simulink model "sampleModel1927"  (R2023a)
settings: Solver=VariableStepAuto  StartTime=0.0  StopTime=10.0  RelTol=1e-3
libraries: hdlsllib x7, simulink x2
settings Model: Creator=user1  LastModifiedBy=user1

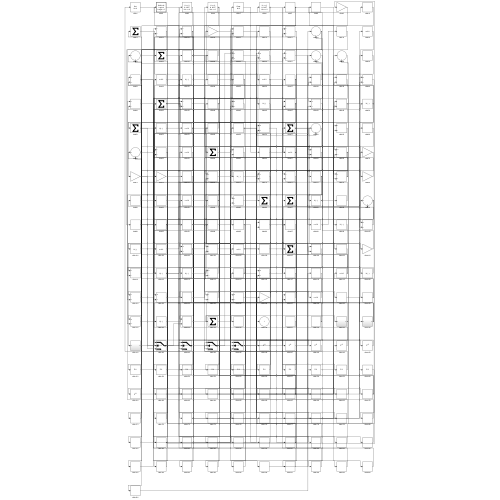
[thumbnail: Simulink's stored preview of the top-level diagram]
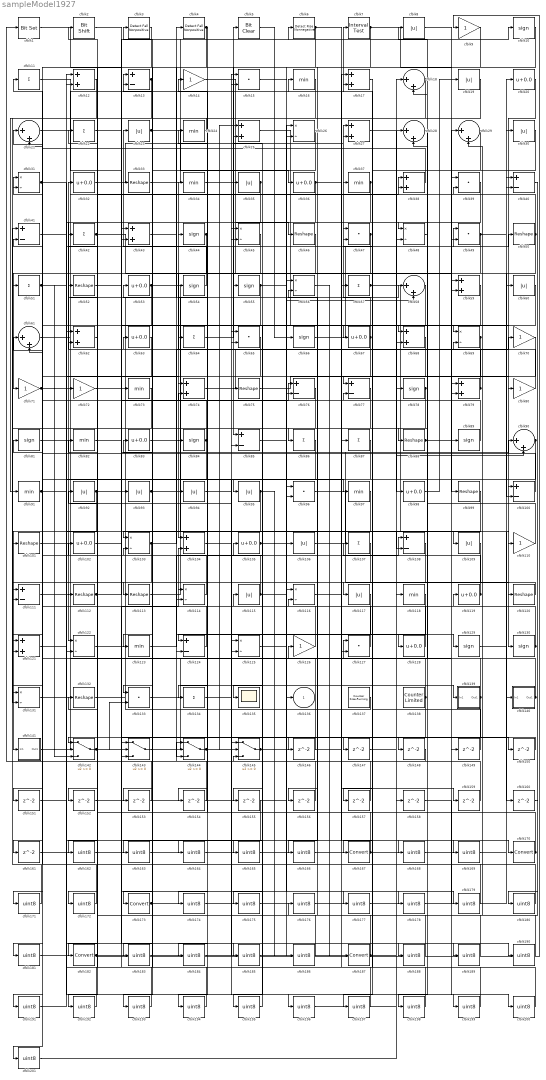
== system sampleModel1927 ==
  cfblk1 : simulink/Logic and Bit Operations/Bit Set  iBit=0
      settings: LibrarySourceBlock=|
      | hdlsllib/Logic and Bit
      | Operations/Bit Set
  cfblk{10,44,54..55,66,78,81,84,89,129..130} (11 alike) : Signum
  cfblk{13,40..41,76..77,85,100,108,111,124} (10 alike) : Sum  Inputs=+-
  cfblk{33,46,50,52,75,88,99,101,112..113,120,132} (12 alike) : Reshape
  cfblk{20,32,36,53,63,67,83,98,102,105,119,128} (12 alike) : Bias  Bias=0.0  SaturateOnIntegerOverflow=off
  cfblk{26,31,45,48,56,69,103,114,116,122,125,131} (12 alike) : Product  Inputs=*/  RndMeth=Zero  SaturateOnIntegerOverflow=on
  cfblk{12,17,25,27,38,43,59,62,68,74,79,104,121} (13 alike) : Sum
  cfblk{8,19,23,30,35,60,92..95,106,109,115,117} (14 alike) : Abs  SaturateOnIntegerOverflow=off
  cfblk{11,22,42,51,57,64,86..87,107,134} (10 alike) : Sum  Inputs=+
  cfblk{9,14,70..72,80,110,126} (8 alike) : Gain
  cfblk{16,24,34,37,73,82,91,97,118,123} (10 alike) : MinMax
  cfblk{15,39,47,49,65,96,127,133} (8 alike) : DotProduct  OutDataTypeStr=Inherit: Inherit via internal rule
  cfblk135 : Scope
  cfblk137 : hdlsllib/Sources/Counter Free-Running  NumBits=16  tsamp=-1
  cfblk138 : hdlsllib/Sources/Counter Limited  uplimit=7  tsamp=-1
  cfblk139 : Subsystem
      settings: LibrarySourceBlock=|
      | hdlsllib/Ports &
      | Subsystems/Subsystem
  cfblk140 : Subsystem
      settings: LibrarySourceBlock=|
      | hdlsllib/Ports &
      | Subsystems/Subsystem
  cfblk141 : Subsystem
      settings: LibrarySourceBlock=|
      | hdlsllib/Ports &
      | Subsystems/Subsystem
  cfblk{142..145} (4 alike) : Switch  SaturateOnIntegerOverflow=off  InputSameDT=off
  cfblk{146..161} (16 alike) : Delay  SampleTime=1
  cfblk{162..166,168..169,171..172,174..181,183..186,188..201} (35 alike) : DataTypeConversion  OutDataTypeStr=uint8  SaturateOnIntegerOverflow=off  RndMeth=Floor
  cfblk{167,170,173,182,187} (5 alike) : DataTypeConversion  SaturateOnIntegerOverflow=off  RndMeth=Floor
  cfblk{18,21,28..29,58,61,90} (7 alike) : Sum  Inputs=|++
  cfblk2 : hdlsllib/Logic and Bit Operations/Bit Shift  mode=Shift Left Logical  N=0
  cfblk3 : hdlsllib/Logic and Bit Operations/Detect Fall Nonpositive  vinit=0  OutDataTypeStr=boolean
  cfblk4 : hdlsllib/Logic and Bit Operations/Detect Fall Nonpositive  vinit=0  OutDataTypeStr=boolean
  cfblk5 : simulink/Logic and Bit Operations/Bit Clear  iBit=0
      settings: LibrarySourceBlock=|
      | hdlsllib/Logic and Bit
      | Operations/Bit Clear
  cfblk6 : hdlsllib/Logic and Bit Operations/Detect Rise Nonnegative  vinit=0  OutDataTypeStr=boolean
  cfblk7 : hdlsllib/Logic and Bit Operations/Interval Test  IntervalClosedRight=on  uplimit=0.5  IntervalClosedLeft=on  lowlimit=-0.5  OutDataTypeStr=boolean
  cfblk136 : Outport  VectorParamsAs1DForOutWhenUnconnected=off
  wires:
  cfblk20/1 -> cfblk130/1
  cfblk5/1 -> cfblk66/1
  cfblk98/1 -> cfblk19/1
  cfblk78/1 -> cfblk86/1, cfblk157/1
  cfblk54/1 -> cfblk23/1
  cfblk32/1 -> cfblk27/1
  cfblk26/1 -> cfblk173/1
  cfblk24/1 -> cfblk91/1
  cfblk33/1 -> cfblk10/1
  cfblk64/1 -> cfblk5/1
  cfblk9/1 -> cfblk85/1
  cfblk126/1 -> cfblk115/1
  cfblk133/1 -> cfblk139/1(In1)
  cfblk137/1 -> cfblk53/1
  cfblk67/1 -> cfblk27/2, cfblk165/1
  cfblk112/1 -> cfblk90/1, cfblk147/1
  cfblk122/1 -> cfblk34/1
  cfblk57/1 -> cfblk110/1, cfblk90/2
  cfblk66/1 -> cfblk50/1
  cfblk113/1 -> cfblk55/1
  cfblk45/1 -> cfblk104/1
  cfblk111/1 -> cfblk16/1
  cfblk132/1 -> cfblk127/1
  cfblk141/1(Out1) -> cfblk47/1
  cfblk25/1 -> cfblk100/1
  cfblk29/1 -> cfblk167/1
  cfblk14/1 -> cfblk46/1
  cfblk145/1 -> cfblk57/1, cfblk175/1, cfblk178/1
  cfblk8/1 -> cfblk79/1
  cfblk36/1 -> cfblk122/1, cfblk159/1
  cfblk142/1 -> cfblk133/2, cfblk114/1, cfblk177/1
  cfblk81/1 -> cfblk58/1
  cfblk80/1 -> cfblk32/1
  cfblk96/1 -> cfblk120/1
  cfblk120/1 -> cfblk117/1
  cfblk100/1 -> cfblk31/1
  cfblk46/1 -> cfblk124/1
  cfblk123/1 -> cfblk108/1
  cfblk92/1 -> cfblk141/1(In1), cfblk76/1
  cfblk143/1 -> cfblk39/1
  cfblk34/1 -> cfblk78/1
  cfblk116/1 -> cfblk87/1
  cfblk131/1 -> cfblk85/2
  cfblk127/1 -> cfblk104/2
  cfblk1/1 -> cfblk93/1
  cfblk124/1 -> cfblk2/1
  cfblk103/1 -> cfblk70/1, cfblk121/2
  cfblk37/1 -> cfblk112/1, cfblk166/1
  cfblk95/1 -> cfblk106/1, cfblk154/1
  cfblk85/1 -> cfblk136/1
  cfblk84/1 -> cfblk21/1, cfblk111/1
  cfblk106/1 -> cfblk60/1
  cfblk71/1 -> cfblk37/1, cfblk142/3
  cfblk138/1 -> cfblk52/1, cfblk42/1, cfblk143/3
  cfblk65/1 -> cfblk182/1
  cfblk27/1 -> cfblk98/1
  cfblk128/1 -> cfblk116/2
  cfblk47/1 -> cfblk71/1, cfblk64/1
  cfblk144/1 -> cfblk25/1, cfblk196/1
  cfblk93/1 -> cfblk145/1, cfblk94/1
  cfblk61/1 -> cfblk4/1
  cfblk75/1 -> cfblk80/1
  cfblk21/1 -> cfblk7/1
  cfblk79/1 -> cfblk44/1, cfblk75/1
  cfblk53/1 -> cfblk140/1(In1), cfblk143/2, cfblk13/2
  cfblk39/1 -> cfblk122/2
  cfblk90/1 -> cfblk125/2, cfblk194/1
  cfblk31/1 -> cfblk74/1, cfblk188/1
  cfblk49/1 -> cfblk30/1, cfblk68/2
  cfblk50/1 -> cfblk121/1, cfblk22/1, cfblk38/2, cfblk100/2
  cfblk68/1 -> cfblk77/1
  cfblk35/1 -> cfblk123/1, cfblk183/1
  cfblk114/1 -> cfblk81/1
  cfblk77/1 -> cfblk103/1
  cfblk2/1 -> cfblk43/1
  cfblk43/1 -> cfblk69/1
  cfblk11/1 -> cfblk73/1
  cfblk18/1 -> cfblk111/2, cfblk151/1
  cfblk104/1 -> cfblk128/1
  cfblk69/1 -> cfblk95/1, cfblk114/2
  cfblk83/1 -> cfblk108/2
  cfblk42/1 -> cfblk79/2, cfblk76/2
  cfblk13/1 -> cfblk131/1, cfblk43/2
  cfblk109/1 -> cfblk135/1
  cfblk76/1 -> cfblk131/2
  cfblk105/1 -> cfblk150/1, cfblk186/1
  cfblk12/1 -> cfblk51/1
  cfblk102/1 -> cfblk6/1
  cfblk52/1 -> cfblk38/1
  cfblk63/1 -> cfblk101/1
  cfblk44/1 -> cfblk14/1, cfblk191/1
  cfblk23/1 -> cfblk36/1, cfblk129/1
  cfblk86/1 -> cfblk144/3
  cfblk41/1 -> cfblk170/1
  cfblk89/1 -> cfblk61/1
  cfblk10/1 -> cfblk96/2
  cfblk48/1 -> cfblk88/1
  cfblk110/1 -> cfblk28/2
  cfblk51/1 -> cfblk109/1, cfblk142/2
  cfblk115/1 -> cfblk24/1, cfblk169/1
  cfblk91/1 -> cfblk49/1, cfblk97/1
  cfblk4/1 -> cfblk84/1, cfblk163/1
  cfblk117/1 -> cfblk134/1
  cfblk101/1 -> cfblk45/1
  cfblk97/1 -> cfblk133/1
  cfblk55/1 -> cfblk68/1, cfblk58/2, cfblk181/1
  cfblk38/1 -> cfblk11/1
  cfblk134/1 -> cfblk45/2
  cfblk16/1 -> cfblk35/1
  cfblk139/1(Out1) -> cfblk63/1, cfblk174/1
  cfblk130/1 -> cfblk31/2, cfblk119/1
  cfblk88/1 -> cfblk89/1, cfblk8/1
  cfblk7/1 -> cfblk99/1, cfblk146/1, cfblk161/1
  cfblk99/1 -> cfblk113/1
  cfblk119/1 -> cfblk77/2, cfblk107/1
  cfblk140/1(Out1) -> cfblk18/2, cfblk13/1, cfblk126/1
  cfblk74/1 -> cfblk69/2
  cfblk56/1 -> cfblk187/1
  cfblk22/1 -> cfblk67/1
  cfblk28/1 -> cfblk48/1
  cfblk6/1 -> cfblk124/2, cfblk168/1
  cfblk146/1 -> cfblk21/2
  cfblk147/1 -> cfblk28/1
  cfblk125/1 -> cfblk148/1
  cfblk148/1 -> cfblk1/1
  cfblk149/1 -> cfblk47/2
  cfblk150/1 -> cfblk142/1
  cfblk151/1 -> cfblk12/2
  cfblk87/1 -> cfblk152/1
  cfblk152/1 -> cfblk116/1
  cfblk108/1 -> cfblk153/1
  cfblk153/1 -> cfblk61/2
  cfblk154/1 -> cfblk144/2
  cfblk60/1 -> cfblk155/1
  cfblk58/1 -> cfblk156/1
  cfblk156/1 -> cfblk144/1
  cfblk157/1 -> cfblk145/2
  cfblk159/1 -> cfblk145/3
  cfblk129/1 -> cfblk160/1
  cfblk161/1 -> cfblk48/2
  cfblk3/1 -> cfblk162/1
  cfblk162/1 -> cfblk20/1
  cfblk163/1 -> cfblk3/1
  cfblk59/1 -> cfblk164/1
  cfblk164/1 -> cfblk127/2
  cfblk165/1 -> cfblk59/1
  cfblk166/1 -> cfblk59/2
  cfblk167/1 -> cfblk74/2, cfblk132/1, cfblk33/1
  cfblk168/1 -> cfblk29/1
  cfblk169/1 -> cfblk29/2
  cfblk170/1 -> cfblk25/2, cfblk54/1
  cfblk73/1 -> cfblk171/1
  cfblk171/1 -> cfblk41/1
  cfblk107/1 -> cfblk172/1
  cfblk172/1 -> cfblk41/2
  cfblk173/1 -> cfblk49/2, cfblk125/1
  cfblk174/1 -> cfblk26/1
  cfblk175/1 -> cfblk26/2
  cfblk40/1 -> cfblk176/1
  cfblk176/1 -> cfblk149/1
  cfblk177/1 -> cfblk40/1
  cfblk178/1 -> cfblk40/2
  cfblk15/1 -> cfblk179/1
  cfblk179/1 -> cfblk92/1
  cfblk160/1 -> cfblk180/1
  cfblk180/1 -> cfblk15/1
  cfblk181/1 -> cfblk15/2
  cfblk182/1 -> cfblk9/1, cfblk96/1
  cfblk183/1 -> cfblk65/1
  cfblk19/1 -> cfblk184/1
  cfblk184/1 -> cfblk65/2
  cfblk82/1 -> cfblk185/1
  cfblk185/1 -> cfblk18/1
  cfblk186/1 -> cfblk82/1
  cfblk187/1 -> cfblk83/1, cfblk102/1
  cfblk188/1 -> cfblk56/1
  cfblk94/1 -> cfblk189/1
  cfblk189/1 -> cfblk56/2
  cfblk72/1 -> cfblk190/1
  cfblk190/1 -> cfblk39/2
  cfblk191/1 -> cfblk72/1
  cfblk62/1 -> cfblk192/1
  cfblk192/1 -> cfblk12/1
  cfblk155/1 -> cfblk193/1
  cfblk193/1 -> cfblk62/1
  cfblk194/1 -> cfblk62/2
  cfblk118/1 -> cfblk195/1
  cfblk195/1 -> cfblk105/1
  cfblk196/1 -> cfblk118/1
  cfblk17/1 -> cfblk197/1
  cfblk197/1 -> cfblk143/1
  cfblk30/1 -> cfblk198/1
  cfblk198/1 -> cfblk17/1
  cfblk121/1 -> cfblk199/1
  cfblk199/1 -> cfblk17/2
  cfblk158/1 -> cfblk200/1
  cfblk200/1 -> cfblk103/2
  cfblk70/1 -> cfblk201/1
  cfblk201/1 -> cfblk158/1

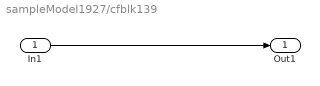
== system sampleModel1927/cfblk139 ==
  In1 : Inport
  Out1 : Outport
  wires:
  In1/1 -> Out1/1

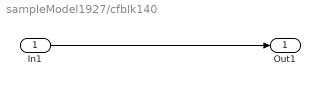
== system sampleModel1927/cfblk140 ==
  In1 : Inport
  Out1 : Outport
  wires:
  In1/1 -> Out1/1

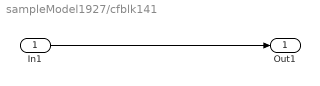
== system sampleModel1927/cfblk141 ==
  In1 : Inport
  Out1 : Outport
  wires:
  In1/1 -> Out1/1
